simulink model "vector"  (R2025b)
settings: Solver=FixedStepAuto  StartTime=0.0  StopTime=30  FixedStep=0.05  RelTol=1e-3
undefined symbols (not defined in the file or in its folder): DiscIntNeverNeededParam
libraries: rllib x1
(part 1 of 2)
settings Model: Creator=heodo  LastModifiedBy=heodo

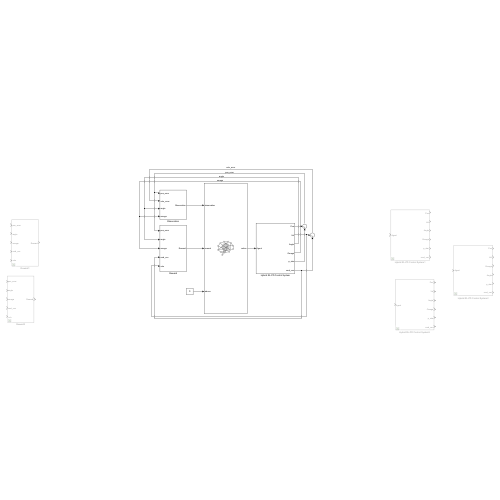
[thumbnail: Simulink's stored preview of the top-level diagram]
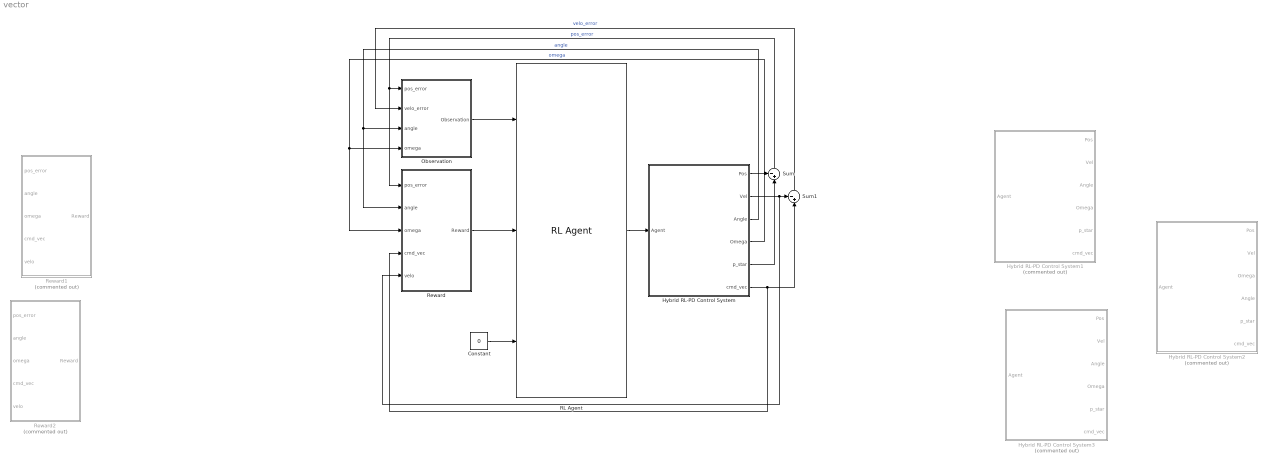
== system vector ==
  Constant : Constant  Value=0
  Hybrid RL-PD Control System : Subsystem
  Hybrid RL-PD Control System1 : Subsystem  Commented=on
  Hybrid RL-PD Control System2 : Subsystem  Commented=on
  Hybrid RL-PD Control System3 : Subsystem  Commented=on
  Observation : Subsystem
  RL Agent : rllib/RL Agent  Agent=agent  ExternalActionAsInput=off  ProvideLastAction=off  ProvideCumRwd=off  TreatAsDirectFeedthrough=on  UseStrictObservationDataTypes=off
  Reward : Subsystem
  Reward1 : Subsystem  Commented=on
  Reward2 : Subsystem  Commented=on
  Sum : Sum  Inputs=-+|
  Sum1 : Sum  Inputs=-+|
  wires:
  Observation/1(Observation) -> RL Agent/1
  Reward/1(Reward) -> RL Agent/2
  RL Agent/1 -> Hybrid RL-PD Control System/1(Agent)
  Hybrid RL-PD Control System/1(Pos) -> Sum/1
  Hybrid RL-PD Control System/5(p_star) -> Sum/2
  Sum/1 -> Reward/1(pos_error), Observation/1(pos_error)  "pos_error"
  Hybrid RL-PD Control System/2(Vel) -> Reward/5(velo), Sum1/1
  Hybrid RL-PD Control System/6(cmd_vec) -> Sum1/2, Reward/4(cmd_vec)
  Sum1/1 -> Observation/2(velo_error)  "velo_error"
  Hybrid RL-PD Control System/3(Angle) -> Observation/3(angle), Reward/2(angle)  "angle"
  Hybrid RL-PD Control System/4(Omega) -> Observation/4(omega), Reward/3(omega)  "omega"
  Constant/1 -> RL Agent/3

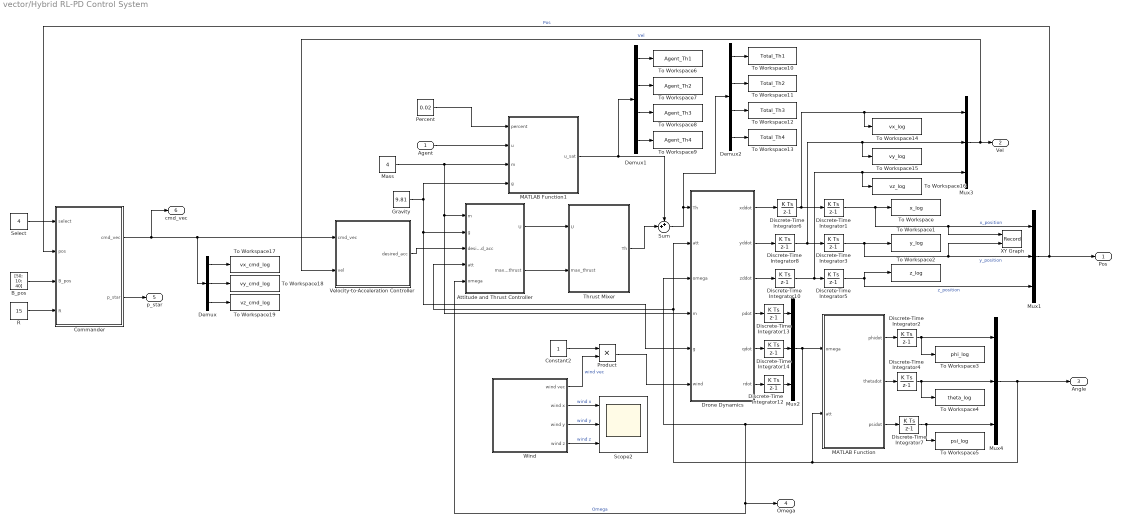
== system vector/Hybrid RL-PD Control System ==
  Agent : Inport
  Attitude and Thrust Controller : MATLAB Function  TreatAsAtomicUnit=on
  B_pos : Constant  Value=[50; 10; 40]
  Commander : MATLAB Function  TreatAsAtomicUnit=on
  Constant2 : Constant
  Demux : Demux  Outputs=3
  Demux1 : Demux
  Demux2 : Demux
  Discrete-Time Integrator{1..4,6..8,10,12..14} (11 alike) : DiscreteIntegrator  SampleTime=-1  ICPrevOutput=DiscIntNeverNeededParam  ICPrevScaledInput=DiscIntNeverNeededParam
  Discrete-Time Integrator5 : DiscreteIntegrator  InitialCondition=25  SampleTime=-1  ICPrevOutput=DiscIntNeverNeededParam  ICPrevScaledInput=DiscIntNeverNeededParam
  Drone Dynamics : MATLAB Function  TreatAsAtomicUnit=on
  Gravity : Constant  Value=9.81
  MATLAB Function : MATLAB Function  TreatAsAtomicUnit=on
  MATLAB Function1 : MATLAB Function  TreatAsAtomicUnit=on
  Mass : Constant  Value=4
  Mux{1..4} (4 alike) : Mux  Inputs=3
  Percent : Constant  Value=0.02
  Product : Product
  R : Constant  Value=15
  Scope2 : Scope  NumInputPorts=3
      settings: ActiveDisplayYMinimum=-12.935318443726832  ActiveDisplayYMaximum=12.935318443726839  DataLoggingVariableName=ScopeData2
  Select : Constant  Value=4
  Sum : Sum  Inputs=++|
  Thrust Mixer : MATLAB Function  TreatAsAtomicUnit=on
  To Workspace : ToWorkspace  VariableName=x_log  SaveFormat=Timeseries  SampleTime=-1
  To Workspace1 : ToWorkspace  VariableName=y_log  SaveFormat=Timeseries  SampleTime=-1
  To Workspace10 : ToWorkspace  VariableName=Total_Th1  SaveFormat=Timeseries  SampleTime=-1
  To Workspace11 : ToWorkspace  VariableName=Total_Th2  SaveFormat=Timeseries  SampleTime=-1
  To Workspace12 : ToWorkspace  VariableName=Total_Th3  SaveFormat=Timeseries  SampleTime=-1
  To Workspace13 : ToWorkspace  VariableName=Total_Th4  SaveFormat=Timeseries  SampleTime=-1
  To Workspace14 : ToWorkspace  VariableName=vx_log  SaveFormat=Timeseries  SampleTime=-1
  To Workspace15 : ToWorkspace  VariableName=vy_log  SaveFormat=Timeseries  SampleTime=-1
  To Workspace16 : ToWorkspace  VariableName=vz_log  SaveFormat=Timeseries  SampleTime=-1
  To Workspace17 : ToWorkspace  VariableName=vx_cmd_log  SaveFormat=Timeseries  SampleTime=-1
  To Workspace18 : ToWorkspace  VariableName=vy_cmd_log  SaveFormat=Timeseries  SampleTime=-1
  To Workspace19 : ToWorkspace  VariableName=vz_cmd_log  SaveFormat=Timeseries  SampleTime=-1
  To Workspace2 : ToWorkspace  VariableName=z_log  SaveFormat=Timeseries  SampleTime=-1
  To Workspace3 : ToWorkspace  VariableName=phi_log  SaveFormat=Timeseries  SampleTime=-1
  To Workspace4 : ToWorkspace  VariableName=theta_log  SaveFormat=Timeseries  SampleTime=-1
  To Workspace5 : ToWorkspace  VariableName=psi_log  SaveFormat=Timeseries  SampleTime=-1
  To Workspace6 : ToWorkspace  VariableName=Agent_Th1  SaveFormat=Timeseries  SampleTime=-1
  To Workspace7 : ToWorkspace  VariableName=Agent_Th2  SaveFormat=Timeseries  SampleTime=-1
  To Workspace8 : ToWorkspace  VariableName=Agent_Th3  SaveFormat=Timeseries  SampleTime=-1
  To Workspace9 : ToWorkspace  VariableName=Agent_Th4  SaveFormat=Timeseries  SampleTime=-1
  Velocity-to-Acceleration Controller : MATLAB Function  TreatAsAtomicUnit=on
  Wind : Subsystem
  XY Graph : Record  NumPorts=2.0  FileSettingsInternal="{\"entries\":[{\"content\":{\"excelSettings\":{\"content\":{},\"type\":\"Streamout.ExcelSettings\"},\"parquetSettings\":{\"content\":{},\"type\":\"Streamout.ParquetSettings\"}},\"type\":\"Streamout.FileSettingStorage\",\"uuid\":\"\"}],\"packageUris\":[\"http:\\/\\/schema.mathworks.com\\/mf0\\/streamout_blocks\\/R2020a\"],\"version\":\"1.0\"}"  FrameSettings=[0, 0]  Layout=[1 1]  SignalsInternal="{\"entries\":[{\"content\":{\"signals\":[{\"content\":{\"blockPath\":[],\"dimensions\":[1],\"domain\":\"\",\"lineColor\":\"#a2142f\",\"plots\":[ 1 ],\"port\":1,\"signalID\":1,\"signalName\":\"x_position\"},\"type\":\"RecordBlkView.Signal\",\"uuid\":\"\"},{\"content\":{\"blockPath\":[],\"dimensions\":[1],\"domain\":\"\",\"lineColor\":\"#139fff\",\"plots\":[ 1 ],\"port\":2,\"signalID\":2,\"signalName\":\"y_position\"},\"type\":\"RecordBlkView.Signal\",\"uuid\":\"\"}]},\"type\":\"RecordBlkView.InputSignals\",\"uuid\":\"\"}],\"packageUris\":[\"http:\\/\\/schema.mathworks.com\\/mf0\\/streamout_blocks\\/R2020a\"],\"version\":\"1.0\"}"  VisualizationBindings="{\"xyplotplugin\":{\"info\":[{\"series\":[{\"bindingParametersList\":[{\"parameter\":\"X-Axis\",\"signalID\":1,\"signalName\":\"x_position\"},{\"parameter\":\"Y-Axis\",\"signalID\":2,\"signalName\":\"y_position\"}],\"seriesID\":0}],\"subplotID\":1}]}}"  CompatibilityTag=XY
  Pos : Outport
  Vel : Outport  Port=2
  Angle : Outport  Port=3
  Omega : Outport  Port=4
  p_star : Outport  Port=5
  cmd_vec : Outport  Port=6
  wires:
  Velocity-to-Acceleration Controller/1(desired_acc) -> Attitude and Thrust Controller/3(desired_acc)
  Gravity/1 -> MATLAB Function1/4(g), Attitude and Thrust Controller/2(g), Drone Dynamics/5(g)
  Mass/1 -> Attitude and Thrust Controller/1(m), Drone Dynamics/4(m), MATLAB Function1/3(m)
  Attitude and Thrust Controller/1(U) -> Thrust Mixer/1(U)
  Attitude and Thrust Controller/2(max_thrust) -> Thrust Mixer/2(max_thrust)
  Mux4/1 -> MATLAB Function/2(att), Drone Dynamics/2(att), Attitude and Thrust Controller/4(att), Angle/1
  Discrete-Time Integrator5/1 -> To Workspace2/1, Mux1/3  "z_position"
  Discrete-Time Integrator1/1 -> XY Graph/1, Mux1/1, To Workspace/1  "x_position"
  Discrete-Time Integrator3/1 -> To Workspace1/1, XY Graph/2, Mux1/2  "y_position"
  Mux1/1 -> Pos/1, Commander/2(pos)  "Pos"
  Thrust Mixer/1(Th) -> Sum/2
  Sum/1 -> Demux2/1, Drone Dynamics/1(Th)
  Mux3/1 -> Vel/1, Velocity-to-Acceleration Controller/2(vel)  "Vel"
  Mux2/1 -> MATLAB Function/1(omega), Drone Dynamics/3(omega), Attitude and Thrust Controller/5(omega), Omega/1  "Omega"
  Demux1/1 -> To Workspace6/1
  Demux1/4 -> To Workspace9/1
  Demux1/3 -> To Workspace8/1
  Demux1/2 -> To Workspace7/1
  Demux2/3 -> To Workspace12/1
  Demux2/4 -> To Workspace13/1
  Demux2/2 -> To Workspace11/1
  Demux2/1 -> To Workspace10/1
  R/1 -> Commander/4(R)
  Select/1 -> Commander/1(select)
  B_pos/1 -> Commander/3(B_pos)
  Commander/1(cmd_vec) -> cmd_vec/1, Demux/1, Velocity-to-Acceleration Controller/1(cmd_vec)
  Commander/2(p_star) -> p_star/1
  Wind/2(wind x) -> Scope2/1  "wind x"
  Wind/3(wind y) -> Scope2/2  "wind y"
  Wind/4(wind z) -> Scope2/3  "wind z"
  Wind/1(wind vec) -> Product/2  "wind vec"
  Constant2/1 -> Product/1
  Product/1 -> Drone Dynamics/6(wind)
  Drone Dynamics/3(zddot) -> Discrete-Time Integrator10/1
  Drone Dynamics/2(yddot) -> Discrete-Time Integrator8/1
  Drone Dynamics/1(xddot) -> Discrete-Time Integrator6/1
  Discrete-Time Integrator6/1 -> Discrete-Time Integrator1/1, To Workspace14/1, Mux3/1
  Discrete-Time Integrator8/1 -> Discrete-Time Integrator3/1, To Workspace15/1, Mux3/2
  Discrete-Time Integrator10/1 -> To Workspace16/1, Mux3/3, Discrete-Time Integrator5/1
  Discrete-Time Integrator12/1 -> Mux2/3
  Drone Dynamics/6(rdot) -> Discrete-Time Integrator12/1
  Drone Dynamics/5(qdot) -> Discrete-Time Integrator14/1
  Discrete-Time Integrator14/1 -> Mux2/2
  Drone Dynamics/4(pdot) -> Discrete-Time Integrator13/1
  Discrete-Time Integrator13/1 -> Mux2/1
  MATLAB Function/1(phidot) -> Discrete-Time Integrator2/1
  MATLAB Function/2(thetadot) -> Discrete-Time Integrator4/1
  MATLAB Function/3(psidot) -> Discrete-Time Integrator7/1
  Discrete-Time Integrator2/1 -> Mux4/1, To Workspace3/1
  Discrete-Time Integrator4/1 -> To Workspace4/1, Mux4/2
  Discrete-Time Integrator7/1 -> To Workspace5/1, Mux4/3
  Demux/1 -> To Workspace17/1
  Demux/2 -> To Workspace18/1
  Demux/3 -> To Workspace19/1
  Agent/1 -> MATLAB Function1/2(u)
  MATLAB Function1/1(u_sat) -> Sum/1, Demux1/1
  Percent/1 -> MATLAB Function1/1(percent)

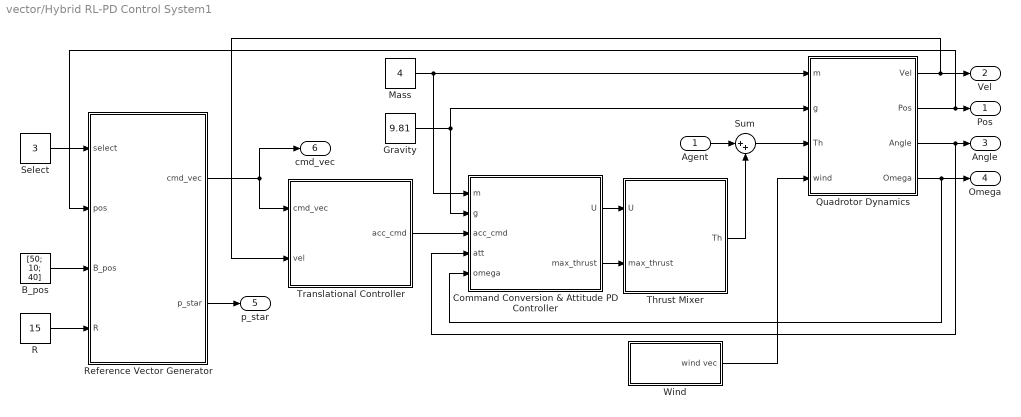
== system vector/Hybrid RL-PD Control System1 ==
  Agent : Inport
  B_pos : Constant  Value=[50; 10; 40]
  Command Conversion & Attitude PD Controller : MATLAB Function  TreatAsAtomicUnit=on
  Gravity : Constant  Value=9.81
  Mass : Constant  Value=4
  Quadrotor Dynamics : Subsystem
  R : Constant  Value=15
  Reference Vector Generator : MATLAB Function  TreatAsAtomicUnit=on
  Select : Constant  Value=3
  Sum : Sum  Inputs=|++
  Thrust Mixer : MATLAB Function  TreatAsAtomicUnit=on
  Translational Controller : MATLAB Function  TreatAsAtomicUnit=on
  Wind : Subsystem
  Pos : Outport
  Vel : Outport  Port=2
  Angle : Outport  Port=3
  Omega : Outport  Port=4
  p_star : Outport  Port=5
  cmd_vec : Outport  Port=6
  wires:
  Translational Controller/1(acc_cmd) -> Command Conversion & Attitude PD Controller/3(acc_cmd)
  Gravity/1 -> Quadrotor Dynamics/2(g), Command Conversion & Attitude PD Controller/2(g)
  Mass/1 -> Command Conversion & Attitude PD Controller/1(m), Quadrotor Dynamics/1(m)
  Command Conversion & Attitude PD Controller/1(U) -> Thrust Mixer/1(U)
  Command Conversion & Attitude PD Controller/2(max_thrust) -> Thrust Mixer/2(max_thrust)
  R/1 -> Reference Vector Generator/4(R)
  Select/1 -> Reference Vector Generator/1(select)
  B_pos/1 -> Reference Vector Generator/3(B_pos)
  Reference Vector Generator/1(cmd_vec) -> cmd_vec/1, Translational Controller/1(cmd_vec)
  Reference Vector Generator/2(p_star) -> p_star/1
  Sum/1 -> Quadrotor Dynamics/3(Th)
  Wind/1(wind vec) -> Quadrotor Dynamics/4(wind)
  Quadrotor Dynamics/1(Vel) -> Vel/1, Translational Controller/2(vel)
  Quadrotor Dynamics/3(Angle) -> Angle/1, Command Conversion & Attitude PD Controller/4(att)
  Quadrotor Dynamics/4(Omega) -> Omega/1, Command Conversion & Attitude PD Controller/5(omega)
  Quadrotor Dynamics/2(Pos) -> Pos/1, Reference Vector Generator/2(pos)
  Agent/1 -> Sum/1
  Thrust Mixer/1(Th) -> Sum/2

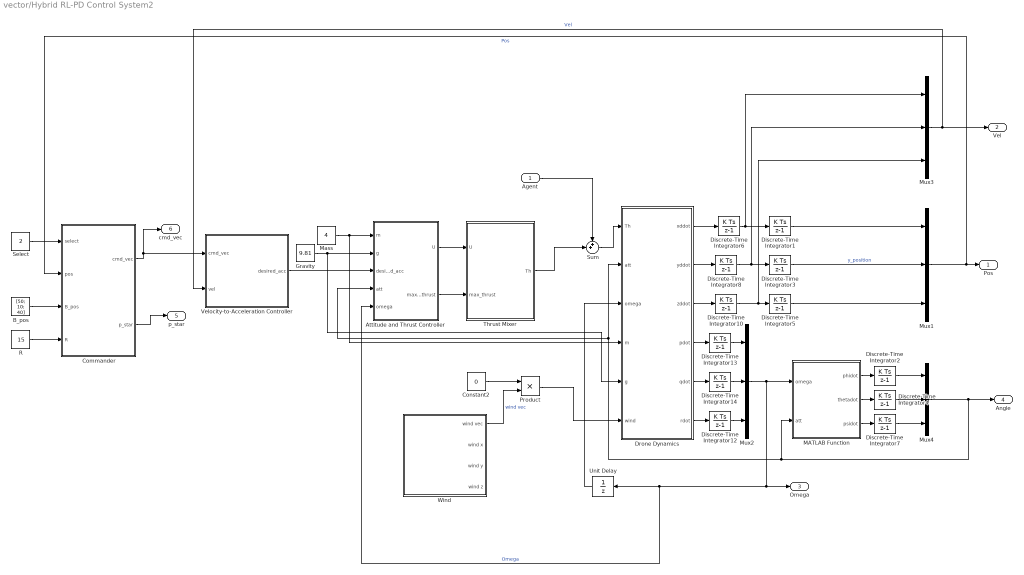
== system vector/Hybrid RL-PD Control System2 ==
  Agent : Inport
  Attitude and Thrust Controller : MATLAB Function  TreatAsAtomicUnit=on
  B_pos : Constant  Value=[50; 10; 40]
  Commander : MATLAB Function  TreatAsAtomicUnit=on
  Constant2 : Constant  Value=0
  Discrete-Time Integrator{1..4,7,12..14} (8 alike) : DiscreteIntegrator  SampleTime=-1  ICPrevOutput=DiscIntNeverNeededParam  ICPrevScaledInput=DiscIntNeverNeededParam
  Discrete-Time Integrator{5..6,8,10} (4 alike) : DiscreteIntegrator  InitialCondition=25  SampleTime=-1  ICPrevOutput=DiscIntNeverNeededParam  ICPrevScaledInput=DiscIntNeverNeededParam
  Drone Dynamics : MATLAB Function  TreatAsAtomicUnit=on
  Gravity : Constant  Value=9.81
  MATLAB Function : MATLAB Function  TreatAsAtomicUnit=on
  Mass : Constant  Value=4
  Mux{1..4} (4 alike) : Mux  Inputs=3
  Product : Product
  R : Constant  Value=15
  Select : Constant  Value=2
  Sum : Sum  Inputs=++|
  Thrust Mixer : MATLAB Function  TreatAsAtomicUnit=on
  Unit Delay : UnitDelay  SampleTime=-1  HasFrameUpgradeWarning=on
  Velocity-to-Acceleration Controller : MATLAB Function  TreatAsAtomicUnit=on
  Wind : Subsystem
  Pos : Outport
  Vel : Outport  Port=2
  Omega : Outport  Port=3
  Angle : Outport  Port=4
  p_star : Outport  Port=5
  cmd_vec : Outport  Port=6
  wires:
  Velocity-to-Acceleration Controller/1(desired_acc) -> Attitude and Thrust Controller/3(desired_acc)
  Gravity/1 -> Attitude and Thrust Controller/2(g), Drone Dynamics/5(g)
  Mass/1 -> Attitude and Thrust Controller/1(m), Drone Dynamics/4(m)
  Attitude and Thrust Controller/1(U) -> Thrust Mixer/1(U)
  Attitude and Thrust Controller/2(max_thrust) -> Thrust Mixer/2(max_thrust)
  Mux4/1 -> Angle/1, Drone Dynamics/2(att), Attitude and Thrust Controller/4(att), MATLAB Function/2(att)
  Discrete-Time Integrator5/1 -> Mux1/3
  Discrete-Time Integrator1/1 -> Mux1/1
  Discrete-Time Integrator3/1 -> Mux1/2  "y_position"
  Mux1/1 -> Pos/1, Commander/2(pos)  "Pos"
  Thrust Mixer/1(Th) -> Sum/2
  Sum/1 -> Drone Dynamics/1(Th)
  Mux3/1 -> Velocity-to-Acceleration Controller/2(vel), Vel/1  "Vel"
  Mux2/1 -> Attitude and Thrust Controller/5(omega), Unit Delay/1, Omega/1, MATLAB Function/1(omega)  "Omega"
  Agent/1 -> Sum/1
  R/1 -> Commander/4(R)
  Select/1 -> Commander/1(select)
  B_pos/1 -> Commander/3(B_pos)
  Commander/1(cmd_vec) -> cmd_vec/1, Velocity-to-Acceleration Controller/1(cmd_vec)
  Commander/2(p_star) -> p_star/1
  Wind/1(wind vec) -> Product/2  "wind vec"
  Constant2/1 -> Product/1
  Product/1 -> Drone Dynamics/6(wind)
  Drone Dynamics/3(zddot) -> Discrete-Time Integrator10/1
  Drone Dynamics/2(yddot) -> Discrete-Time Integrator8/1
  Drone Dynamics/1(xddot) -> Discrete-Time Integrator6/1
  Discrete-Time Integrator6/1 -> Discrete-Time Integrator1/1, Mux3/1
  Discrete-Time Integrator8/1 -> Discrete-Time Integrator3/1, Mux3/2
  Discrete-Time Integrator10/1 -> Mux3/3, Discrete-Time Integrator5/1
  Discrete-Time Integrator12/1 -> Mux2/3
  Drone Dynamics/6(rdot) -> Discrete-Time Integrator12/1
  Drone Dynamics/5(qdot) -> Discrete-Time Integrator14/1
  Discrete-Time Integrator14/1 -> Mux2/2
  Drone Dynamics/4(pdot) -> Discrete-Time Integrator13/1
  Discrete-Time Integrator13/1 -> Mux2/1
  Unit Delay/1 -> Drone Dynamics/3(omega)
  MATLAB Function/1(phidot) -> Discrete-Time Integrator2/1
  MATLAB Function/2(thetadot) -> Discrete-Time Integrator4/1
  MATLAB Function/3(psidot) -> Discrete-Time Integrator7/1
  Discrete-Time Integrator2/1 -> Mux4/1
  Discrete-Time Integrator4/1 -> Mux4/2
  Discrete-Time Integrator7/1 -> Mux4/3

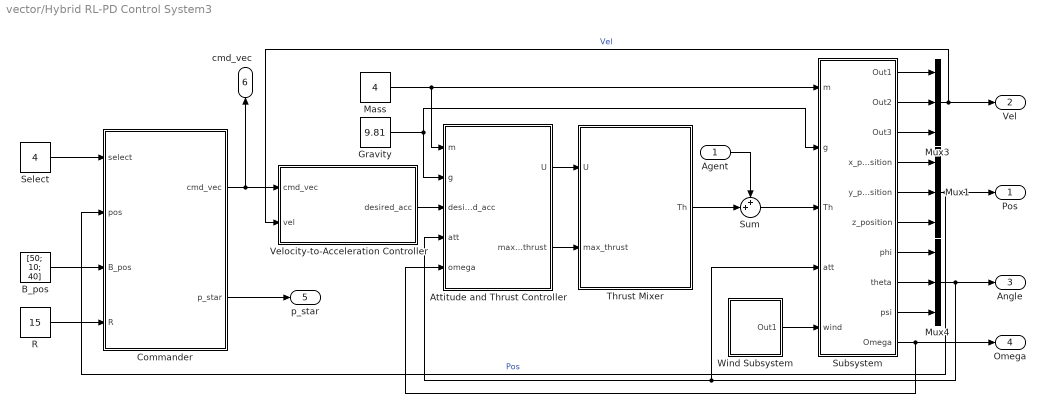
== system vector/Hybrid RL-PD Control System3 ==
  Agent : Inport
  Attitude and Thrust Controller : MATLAB Function  TreatAsAtomicUnit=on
  B_pos : Constant  Value=[50; 10; 40]
  Commander : MATLAB Function  TreatAsAtomicUnit=on
  Gravity : Constant  Value=9.81
  Mass : Constant  Value=4
  Mux1 : Mux  Inputs=3
  Mux3 : Mux  Inputs=3
  Mux4 : Mux  Inputs=3
  R : Constant  Value=15
  Select : Constant  Value=4
  Subsystem : Subsystem
  Sum : Sum  Inputs=++|
  Thrust Mixer : MATLAB Function  TreatAsAtomicUnit=on
  Velocity-to-Acceleration Controller : MATLAB Function  TreatAsAtomicUnit=on
  Wind Subsystem : Subsystem
  Pos : Outport
  Vel : Outport  Port=2
  Angle : Outport  Port=3
  Omega : Outport  Port=4
  p_star : Outport  Port=5
  cmd_vec : Outport  Port=6
  wires:
  Velocity-to-Acceleration Controller/1(desired_acc) -> Attitude and Thrust Controller/3(desired_acc)
  Gravity/1 -> Attitude and Thrust Controller/2(g), Subsystem/2(g)
  Mass/1 -> Attitude and Thrust Controller/1(m), Subsystem/1(m)
  Attitude and Thrust Controller/1(U) -> Thrust Mixer/1(U)
  Attitude and Thrust Controller/2(max_thrust) -> Thrust Mixer/2(max_thrust)
  Mux4/1 -> Angle/1, Attitude and Thrust Controller/4(att), Subsystem/4(att)
  Mux1/1 -> Pos/1, Commander/2(pos)  "Pos"
  Thrust Mixer/1(Th) -> Sum/2
  Mux3/1 -> Vel/1, Velocity-to-Acceleration Controller/2(vel)  "Vel"
  Agent/1 -> Sum/1
  R/1 -> Commander/4(R)
  Select/1 -> Commander/1(select)
  B_pos/1 -> Commander/3(B_pos)
  Commander/1(cmd_vec) -> Velocity-to-Acceleration Controller/1(cmd_vec), cmd_vec/1
  Commander/2(p_star) -> p_star/1
  Subsystem/10(Omega) -> Attitude and Thrust Controller/5(omega), Omega/1
  Sum/1 -> Subsystem/3(Th)
  Wind Subsystem/1(Out1) -> Subsystem/5(wind)
  Subsystem/1(Out1) -> Mux3/1
  Subsystem/2(Out2) -> Mux3/2
  Subsystem/3(Out3) -> Mux3/3
  Subsystem/4(x_position) -> Mux1/1
  Subsystem/5(y_position) -> Mux1/2
  Subsystem/6(z_position) -> Mux1/3
  Subsystem/7(phi) -> Mux4/1
  Subsystem/8(theta) -> Mux4/2
  Subsystem/9(psi) -> Mux4/3

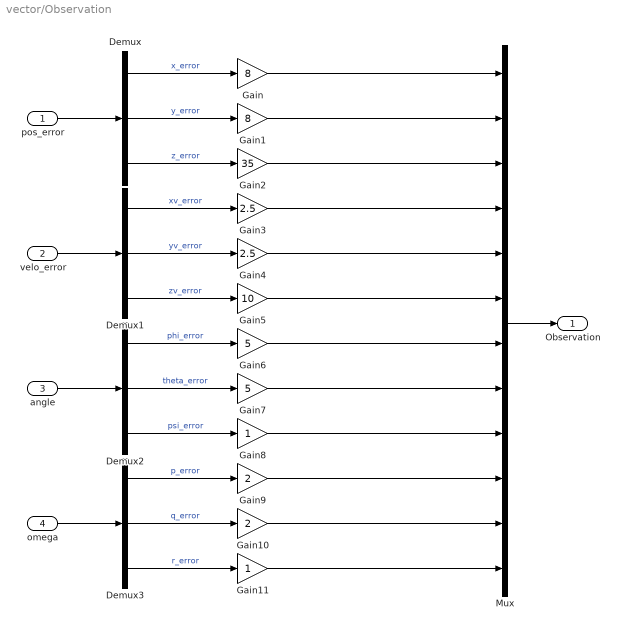
== system vector/Observation ==
  pos_error : Inport
  velo_error : Inport  Port=2
  angle : Inport  Port=3
  omega : Inport  Port=4
  Demux{,1..3} (4 alike) : Demux  Outputs=3
  Gain : Gain  Gain=8
  Gain1 : Gain  Gain=8
  Gain10 : Gain  Gain=2
  Gain11 : Gain
  Gain2 : Gain  Gain=35
  Gain3 : Gain  Gain=2.5
  Gain4 : Gain  Gain=2.5
  Gain5 : Gain  Gain=10
  Gain6 : Gain  Gain=5
  Gain7 : Gain  Gain=5
  Gain8 : Gain
  Gain9 : Gain  Gain=2
  Mux : Mux  Inputs=12
  Observation : Outport
  wires:
  Mux/1 -> Observation/1
  Demux/1 -> Gain/1  "x_error"
  Demux/2 -> Gain1/1  "y_error"
  Demux/3 -> Gain2/1  "z_error"
  Demux1/2 -> Gain4/1  "yv_error"
  Demux1/1 -> Gain3/1  "xv_error"
  Demux1/3 -> Gain5/1  "zv_error"
  Demux2/2 -> Gain7/1  "theta_error"
  Demux2/1 -> Gain6/1  "phi_error"
  Demux2/3 -> Gain8/1  "psi_error"
  Demux3/2 -> Gain10/1  "q_error"
  Demux3/1 -> Gain9/1  "p_error"
  Demux3/3 -> Gain11/1  "r_error"
  omega/1 -> Demux3/1
  angle/1 -> Demux2/1
  velo_error/1 -> Demux1/1
  pos_error/1 -> Demux/1
  Gain/1 -> Mux/1
  Gain1/1 -> Mux/2
  Gain2/1 -> Mux/3
  Gain3/1 -> Mux/4
  Gain4/1 -> Mux/5
  Gain5/1 -> Mux/6
  Gain6/1 -> Mux/7
  Gain7/1 -> Mux/8
  Gain8/1 -> Mux/9
  Gain9/1 -> Mux/10
  Gain10/1 -> Mux/11
  Gain11/1 -> Mux/12

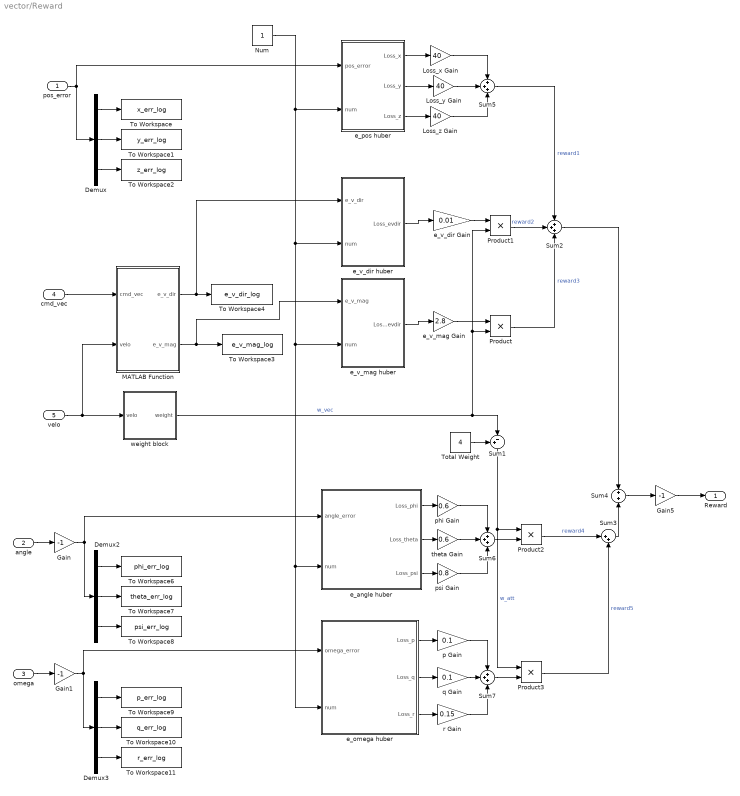
== system vector/Reward ==
  pos_error : Inport
  angle : Inport  Port=2
  omega : Inport  Port=3
  cmd_vec : Inport  Port=4
  velo : Inport  Port=5
  " e_angle huber" : MATLAB Function  TreatAsAtomicUnit=on
  Demux : Demux  Outputs=3
  Demux2 : Demux  Outputs=3
  Demux3 : Demux  Outputs=3
  Gain : Gain  Gain=-1
  Gain1 : Gain  Gain=-1
  Gain5 : Gain  Gain=-1
  Loss_x Gain : Gain  Gain=40
  Loss_y Gain : Gain  Gain=40
  Loss_z Gain : Gain  Gain=40
  MATLAB Function : MATLAB Function  TreatAsAtomicUnit=on
  Num : Constant
  Product{,1..3} (4 alike) : Product
  Sum1 : Sum  Inputs=+-|
  Sum{2,5..7} (4 alike) : Sum  Inputs=+++
  Sum3 : Sum  Inputs=|++
  Sum4 : Sum  Inputs=+|+
  To Workspace : ToWorkspace  VariableName=x_err_log  SaveFormat=Timeseries  SampleTime=-1
  To Workspace1 : ToWorkspace  VariableName=y_err_log  SaveFormat=Timeseries  SampleTime=-1
  To Workspace10 : ToWorkspace  VariableName=q_err_log  SaveFormat=Timeseries  SampleTime=-1
  To Workspace11 : ToWorkspace  VariableName=r_err_log  SaveFormat=Timeseries  SampleTime=-1
  To Workspace2 : ToWorkspace  VariableName=z_err_log  SaveFormat=Timeseries  SampleTime=-1
  To Workspace3 : ToWorkspace  VariableName=e_v_mag_log  SaveFormat=Timeseries  SampleTime=-1
  To Workspace4 : ToWorkspace  VariableName=e_v_dir_log  SaveFormat=Timeseries  SampleTime=-1
  To Workspace6 : ToWorkspace  VariableName=phi_err_log  SaveFormat=Timeseries  SampleTime=-1
  To Workspace7 : ToWorkspace  VariableName=theta_err_log  SaveFormat=Timeseries  SampleTime=-1
  To Workspace8 : ToWorkspace  VariableName=psi_err_log  SaveFormat=Timeseries  SampleTime=-1
  To Workspace9 : ToWorkspace  VariableName=p_err_log  SaveFormat=Timeseries  SampleTime=-1
  Total Weight : Constant  Value=4
  e_omega huber : MATLAB Function  TreatAsAtomicUnit=on
  e_pos huber : MATLAB Function  TreatAsAtomicUnit=on
  e_v_dir Gain : Gain  Gain=0.01
  e_v_dir huber : MATLAB Function  TreatAsAtomicUnit=on
  e_v_mag Gain : Gain  Gain=2.8
  e_v_mag huber : MATLAB Function  TreatAsAtomicUnit=on
  p Gain : Gain  Gain=0.1
  phi Gain : Gain  Gain=0.6
  psi Gain : Gain  Gain=0.8
  q Gain : Gain  Gain=0.1
  r Gain : Gain  Gain=0.15
  theta Gain : Gain  Gain=0.6
  weight block : Subsystem
  Reward : Outport
  wires:
  pos_error/1 -> Demux/1, e_pos huber/1(pos_error)
  Gain5/1 -> Reward/1
  Demux/1 -> To Workspace/1
  Demux/2 -> To Workspace1/1
  Demux/3 -> To Workspace2/1
  MATLAB Function/1(e_v_dir) -> To Workspace4/1, e_v_dir huber/1(e_v_dir)
  Demux2/3 -> To Workspace8/1
  Demux2/1 -> To Workspace6/1
  Demux2/2 -> To Workspace7/1
  angle/1 -> Gain/1
  Demux3/3 -> To Workspace11/1
  Demux3/1 -> To Workspace9/1
  Demux3/2 -> To Workspace10/1
  omega/1 -> Gain1/1
  velo/1 -> MATLAB Function/2(velo), weight block/1(velo)
  Gain/1 -> Demux2/1, " e_angle huber"/1(angle_error)
  Gain1/1 -> Demux3/1, e_omega huber/1(omega_error)
  cmd_vec/1 -> MATLAB Function/1(cmd_vec)
  e_v_mag huber/1(Loss_evdir) -> e_v_mag Gain/1
  e_v_mag Gain/1 -> Product/1
  MATLAB Function/2(e_v_mag) -> To Workspace3/1, e_v_mag huber/1(e_v_mag)
  e_v_dir huber/1(Loss_evdir) -> e_v_dir Gain/1
  e_v_dir Gain/1 -> Product1/1
  Total Weight/1 -> Sum1/1
  Sum1/1 -> Product3/1, Product2/1  "w_att"
  e_pos huber/1(Loss_x) -> Loss_x Gain/1
  Product1/1 -> Sum2/2  "reward2"
  Product/1 -> Sum2/3  "reward3"
  Product2/1 -> Sum3/1  "reward4"
  Product3/1 -> Sum3/2  "reward5"
  Sum3/1 -> Sum4/2
  Sum2/1 -> Sum4/1
  Sum4/1 -> Gain5/1
  weight block/1(weight) -> Product1/2, Product/2, Sum1/2  "w_vec"
  Loss_x Gain/1 -> Sum5/1
  e_pos huber/2(Loss_y) -> Loss_y Gain/1
  Loss_y Gain/1 -> Sum5/2
  e_pos huber/3(Loss_z) -> Loss_z Gain/1
  Loss_z Gain/1 -> Sum5/3
  Sum5/1 -> Sum2/1  "reward1"
  theta Gain/1 -> Sum6/2
  " e_angle huber"/1(Loss_phi) -> phi Gain/1
  " e_angle huber"/2(Loss_theta) -> theta Gain/1
  " e_angle huber"/3(Loss_psi) -> psi Gain/1
  psi Gain/1 -> Sum6/3
  phi Gain/1 -> Sum6/1
  Sum6/1 -> Product2/2
  r Gain/1 -> Sum7/3
  p Gain/1 -> Sum7/1
  Sum7/1 -> Product3/2
  q Gain/1 -> Sum7/2
  e_omega huber/1(Loss_p) -> p Gain/1
  e_omega huber/2(Loss_q) -> q Gain/1
  e_omega huber/3(Loss_r) -> r Gain/1
  Num/1 -> e_pos huber/2(num), e_v_dir huber/2(num), e_v_mag huber/2(num), " e_angle huber"/2(num), e_omega huber/2(num)

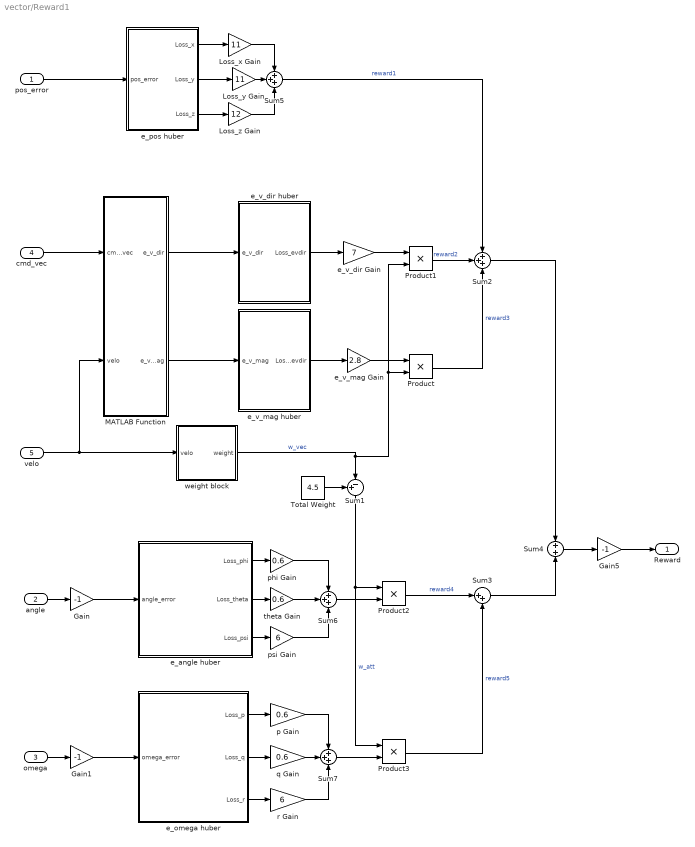
== system vector/Reward1 ==
  pos_error : Inport
  angle : Inport  Port=2
  omega : Inport  Port=3
  cmd_vec : Inport  Port=4
  velo : Inport  Port=5
  " e_angle huber" : MATLAB Function  TreatAsAtomicUnit=on
  Gain : Gain  Gain=-1
  Gain1 : Gain  Gain=-1
  Gain5 : Gain  Gain=-1
  Loss_x Gain : Gain  Gain=11
  Loss_y Gain : Gain  Gain=11
  Loss_z Gain : Gain  Gain=12
  MATLAB Function : MATLAB Function  TreatAsAtomicUnit=on
  Product{,1..3} (4 alike) : Product
  Sum1 : Sum  Inputs=+-|
  Sum{2,5..7} (4 alike) : Sum  Inputs=+++
  Sum3 : Sum  Inputs=|++
  Sum4 : Sum  Inputs=+|+
  Total Weight : Constant  Value=4.5
  e_omega huber : MATLAB Function  TreatAsAtomicUnit=on
  e_pos huber : MATLAB Function  TreatAsAtomicUnit=on
  e_v_dir Gain : Gain  Gain=7
  e_v_dir huber : MATLAB Function  TreatAsAtomicUnit=on
  e_v_mag Gain : Gain  Gain=2.8
  e_v_mag huber : MATLAB Function  TreatAsAtomicUnit=on
  p Gain : Gain  Gain=0.6
  phi Gain : Gain  Gain=0.6
  psi Gain : Gain  Gain=6
  q Gain : Gain  Gain=0.6
  r Gain : Gain  Gain=6
  theta Gain : Gain  Gain=0.6
  weight block : Subsystem
  Reward : Outport
  wires:
  pos_error/1 -> e_pos huber/1(pos_error)
  Gain5/1 -> Reward/1
  MATLAB Function/1(e_v_dir) -> e_v_dir huber/1(e_v_dir)
  angle/1 -> Gain/1
  omega/1 -> Gain1/1
  velo/1 -> weight block/1(velo), MATLAB Function/2(velo)
  Gain/1 -> " e_angle huber"/1(angle_error)
  Gain1/1 -> e_omega huber/1(omega_error)
  cmd_vec/1 -> MATLAB Function/1(cmd_vec)
  e_v_mag huber/1(Loss_evdir) -> e_v_mag Gain/1
  e_v_mag Gain/1 -> Product/1
  MATLAB Function/2(e_v_mag) -> e_v_mag huber/1(e_v_mag)
  e_v_dir huber/1(Loss_evdir) -> e_v_dir Gain/1
  e_v_dir Gain/1 -> Product1/1
  Total Weight/1 -> Sum1/1
  Sum1/1 -> Product3/1, Product2/1  "w_att"
  e_pos huber/1(Loss_x) -> Loss_x Gain/1
  Product1/1 -> Sum2/2  "reward2"
  Product/1 -> Sum2/3  "reward3"
  Product2/1 -> Sum3/1  "reward4"
  Product3/1 -> Sum3/2  "reward5"
  Sum3/1 -> Sum4/2
  Sum2/1 -> Sum4/1
  Sum4/1 -> Gain5/1
  weight block/1(weight) -> Product1/2, Product/2, Sum1/2  "w_vec"
  Loss_x Gain/1 -> Sum5/1
  e_pos huber/2(Loss_y) -> Loss_y Gain/1
  Loss_y Gain/1 -> Sum5/2
  e_pos huber/3(Loss_z) -> Loss_z Gain/1
  Loss_z Gain/1 -> Sum5/3
  Sum5/1 -> Sum2/1  "reward1"
  theta Gain/1 -> Sum6/2
  " e_angle huber"/1(Loss_phi) -> phi Gain/1
  " e_angle huber"/2(Loss_theta) -> theta Gain/1
  " e_angle huber"/3(Loss_psi) -> psi Gain/1
  psi Gain/1 -> Sum6/3
  phi Gain/1 -> Sum6/1
  Sum6/1 -> Product2/2
  r Gain/1 -> Sum7/3
  p Gain/1 -> Sum7/1
  Sum7/1 -> Product3/2
  q Gain/1 -> Sum7/2
  e_omega huber/1(Loss_p) -> p Gain/1
  e_omega huber/2(Loss_q) -> q Gain/1
  e_omega huber/3(Loss_r) -> r Gain/1

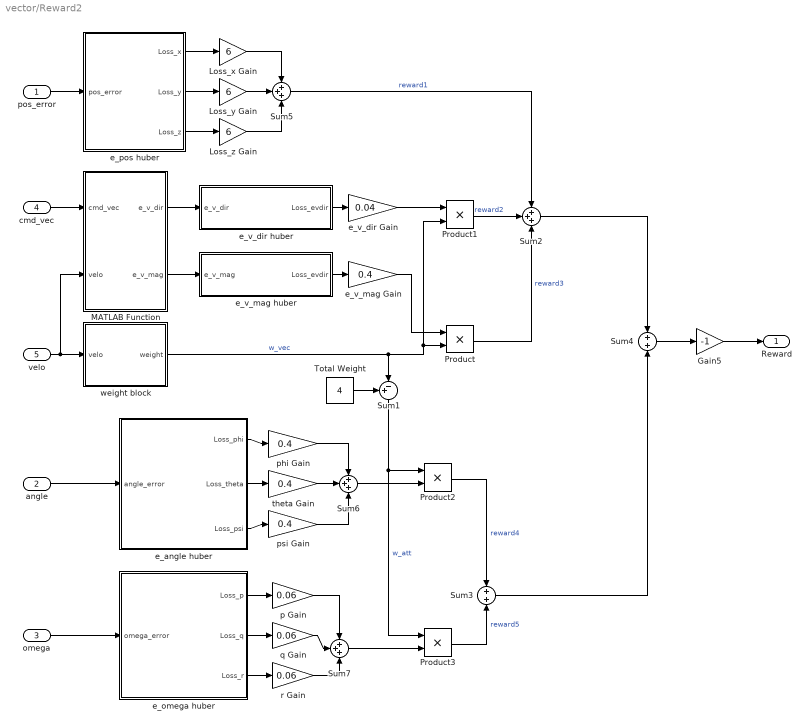
== system vector/Reward2 ==
  pos_error : Inport
  angle : Inport  Port=2
  omega : Inport  Port=3
  cmd_vec : Inport  Port=4
  velo : Inport  Port=5
  " e_angle huber" : MATLAB Function  TreatAsAtomicUnit=on
  Gain5 : Gain  Gain=-1
  Loss_x Gain : Gain  Gain=6
  Loss_y Gain : Gain  Gain=6
  Loss_z Gain : Gain  Gain=6
  MATLAB Function : MATLAB Function  TreatAsAtomicUnit=on
  Product{,1..3} (4 alike) : Product
  Sum1 : Sum  Inputs=+-|
  Sum{2,5..7} (4 alike) : Sum  Inputs=+++
  Sum3 : Sum  Inputs=+|+
  Sum4 : Sum  Inputs=+|+
  Total Weight : Constant  Value=4
  e_omega huber : MATLAB Function  TreatAsAtomicUnit=on
  e_pos huber : MATLAB Function  TreatAsAtomicUnit=on
  e_v_dir Gain : Gain  Gain=0.04
  e_v_dir huber : MATLAB Function  TreatAsAtomicUnit=on
  e_v_mag Gain : Gain  Gain=0.4
  e_v_mag huber : MATLAB Function  TreatAsAtomicUnit=on
  p Gain : Gain  Gain=0.06
  phi Gain : Gain  Gain=0.4
  psi Gain : Gain  Gain=0.4
  q Gain : Gain  Gain=0.06
  r Gain : Gain  Gain=0.06
  theta Gain : Gain  Gain=0.4
  weight block : Subsystem
  Reward : Outport
  wires:
  pos_error/1 -> e_pos huber/1(pos_error)
  Gain5/1 -> Reward/1
  MATLAB Function/1(e_v_dir) -> e_v_dir huber/1(e_v_dir)
  velo/1 -> MATLAB Function/2(velo), weight block/1(velo)
  angle/1 -> " e_angle huber"/1(angle_error)
  omega/1 -> e_omega huber/1(omega_error)
  cmd_vec/1 -> MATLAB Function/1(cmd_vec)
  e_v_mag huber/1(Loss_evdir) -> e_v_mag Gain/1
  e_v_mag Gain/1 -> Product/1
  MATLAB Function/2(e_v_mag) -> e_v_mag huber/1(e_v_mag)
  e_v_dir huber/1(Loss_evdir) -> e_v_dir Gain/1
  e_v_dir Gain/1 -> Product1/1
  Total Weight/1 -> Sum1/1
  Sum1/1 -> Product2/1, Product3/1  "w_att"
  e_pos huber/1(Loss_x) -> Loss_x Gain/1
  Product1/1 -> Sum2/2  "reward2"
  Product/1 -> Sum2/3  "reward3"
  Product2/1 -> Sum3/1  "reward4"
  Product3/1 -> Sum3/2  "reward5"
  Sum3/1 -> Sum4/2
  Sum2/1 -> Sum4/1
  Sum4/1 -> Gain5/1
  weight block/1(weight) -> Product/2, Product1/2, Sum1/2  "w_vec"
  Loss_x Gain/1 -> Sum5/1
  e_pos huber/2(Loss_y) -> Loss_y Gain/1
  Loss_y Gain/1 -> Sum5/2
  e_pos huber/3(Loss_z) -> Loss_z Gain/1
  Loss_z Gain/1 -> Sum5/3
  Sum5/1 -> Sum2/1  "reward1"
  theta Gain/1 -> Sum6/2
  " e_angle huber"/1(Loss_phi) -> phi Gain/1
  " e_angle huber"/2(Loss_theta) -> theta Gain/1
  " e_angle huber"/3(Loss_psi) -> psi Gain/1
  psi Gain/1 -> Sum6/3
  phi Gain/1 -> Sum6/1
  Sum6/1 -> Product2/2
  r Gain/1 -> Sum7/3
  p Gain/1 -> Sum7/1
  Sum7/1 -> Product3/2
  q Gain/1 -> Sum7/2
  e_omega huber/1(Loss_p) -> p Gain/1
  e_omega huber/2(Loss_q) -> q Gain/1
  e_omega huber/3(Loss_r) -> r Gain/1

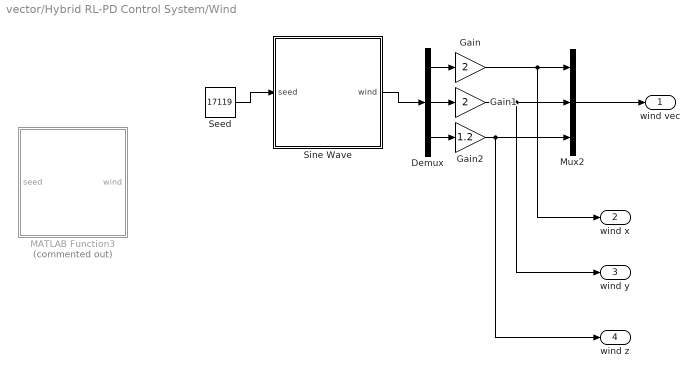
== system vector/Hybrid RL-PD Control System/Wind ==
  Demux : Demux  Outputs=3
  Gain : Gain  Gain=2
  Gain1 : Gain  Gain=2
  Gain2 : Gain  Gain=1.2
  MATLAB Function3 : MATLAB Function  Commented=on  TreatAsAtomicUnit=on
  Mux2 : Mux  Inputs=3
  Seed : Constant  Value=17119
  Sine Wave : MATLAB Function  TreatAsAtomicUnit=on
  wind vec : Outport
  wind x : Outport  Port=2
  wind y : Outport  Port=3
  wind z : Outport  Port=4
  wires:
  Demux/2 -> Gain1/1
  Gain1/1 -> wind y/1, Mux2/2
  Gain2/1 -> wind z/1, Mux2/3
  Demux/1 -> Gain/1
  Demux/3 -> Gain2/1
  Gain/1 -> wind x/1, Mux2/1
  Mux2/1 -> wind vec/1
  Seed/1 -> Sine Wave/1(seed)
  Sine Wave/1(wind) -> Demux/1

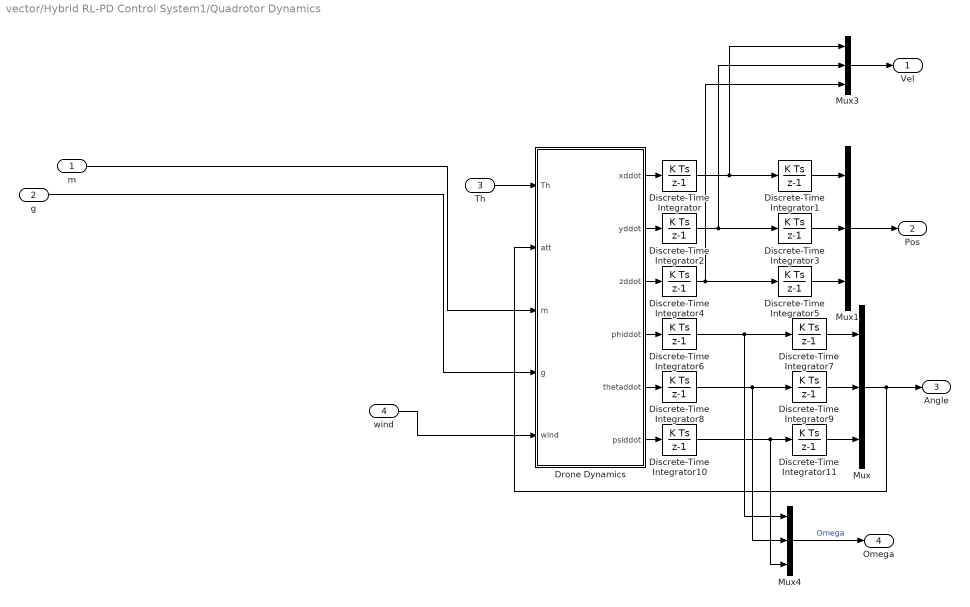
== system vector/Hybrid RL-PD Control System1/Quadrotor Dynamics ==
  m : Inport
  g : Inport  Port=2
  Th : Inport  Port=3
  wind : Inport  Port=4
  Discrete-Time Integrator{,1..4,6..11} (11 alike) : DiscreteIntegrator  SampleTime=-1  ICPrevOutput=DiscIntNeverNeededParam  ICPrevScaledInput=DiscIntNeverNeededParam
  Discrete-Time Integrator5 : DiscreteIntegrator  InitialCondition=25  SampleTime=-1  ICPrevOutput=DiscIntNeverNeededParam  ICPrevScaledInput=DiscIntNeverNeededParam
  Drone Dynamics : MATLAB Function  TreatAsAtomicUnit=on
  Mux{,1,3..4} (4 alike) : Mux  Inputs=3
  Vel : Outport
  Pos : Outport  Port=2
  Angle : Outport  Port=3
  Omega : Outport  Port=4
  wires:
  m/1 -> Drone Dynamics/3(m)
  Mux1/1 -> Pos/1
  Mux3/1 -> Vel/1
  Discrete-Time Integrator/1 -> Discrete-Time Integrator1/1, Mux3/1
  Discrete-Time Integrator5/1 -> Mux1/3
  Discrete-Time Integrator8/1 -> Mux4/2, Discrete-Time Integrator9/1
  Discrete-Time Integrator4/1 -> Discrete-Time Integrator5/1, Mux3/3
  Mux/1 -> Angle/1, Drone Dynamics/2(att)
  g/1 -> Drone Dynamics/4(g)
  Discrete-Time Integrator2/1 -> Discrete-Time Integrator3/1, Mux3/2
  Discrete-Time Integrator7/1 -> Mux/1
  Drone Dynamics/2(yddot) -> Discrete-Time Integrator2/1
  Discrete-Time Integrator3/1 -> Mux1/2
  Discrete-Time Integrator10/1 -> Mux4/3, Discrete-Time Integrator11/1
  Discrete-Time Integrator11/1 -> Mux/3
  Drone Dynamics/6(psiddot) -> Discrete-Time Integrator10/1
  Discrete-Time Integrator1/1 -> Mux1/1
  Discrete-Time Integrator9/1 -> Mux/2
  Drone Dynamics/4(phiddot) -> Discrete-Time Integrator6/1
  Drone Dynamics/5(thetaddot) -> Discrete-Time Integrator8/1
  Discrete-Time Integrator6/1 -> Mux4/1, Discrete-Time Integrator7/1
  Drone Dynamics/3(zddot) -> Discrete-Time Integrator4/1
  Drone Dynamics/1(xddot) -> Discrete-Time Integrator/1
  Mux4/1 -> Omega/1  "Omega"
  wind/1 -> Drone Dynamics/5(wind)
  Th/1 -> Drone Dynamics/1(Th)

== system vector/Hybrid RL-PD Control System1/Wind ==
  Demux : Demux  Outputs=3
  Gain : Gain  Gain=2
  Gain1 : Gain  Gain=2
  Gain2 : Gain  Gain=0.6
  MATLAB Function3 : MATLAB Function  TreatAsAtomicUnit=on
  Mux2 : Mux  Inputs=3
  Seed : Constant  Value=17119
  wind vec : Outport
  wires:
  Demux/2 -> Gain1/1
  Seed/1 -> MATLAB Function3/1(seed)
  Gain1/1 -> Mux2/2
  Gain2/1 -> Mux2/3
  Demux/1 -> Gain/1
  Demux/3 -> Gain2/1
  MATLAB Function3/1(wind) -> Demux/1
  Gain/1 -> Mux2/1
  Mux2/1 -> wind vec/1

== system vector/Hybrid RL-PD Control System2/Wind ==
  Demux : Demux  Outputs=3
  Gain : Gain  Gain=2
  Gain1 : Gain  Gain=2
  Gain2 : Gain  Gain=1.2
  MATLAB Function3 : MATLAB Function  TreatAsAtomicUnit=on
  Mux2 : Mux  Inputs=3
  Seed : Constant  Value=15762
  wind vec : Outport
  wind x : Outport  Port=2
  wind y : Outport  Port=3
  wind z : Outport  Port=4
  wires:
  Demux/2 -> Gain1/1
  Seed/1 -> MATLAB Function3/1(seed)
  Gain1/1 -> wind y/1, Mux2/2
  Gain2/1 -> wind z/1, Mux2/3
  Demux/1 -> Gain/1
  Demux/3 -> Gain2/1
  MATLAB Function3/1(wind) -> Demux/1
  Gain/1 -> wind x/1, Mux2/1
  Mux2/1 -> wind vec/1

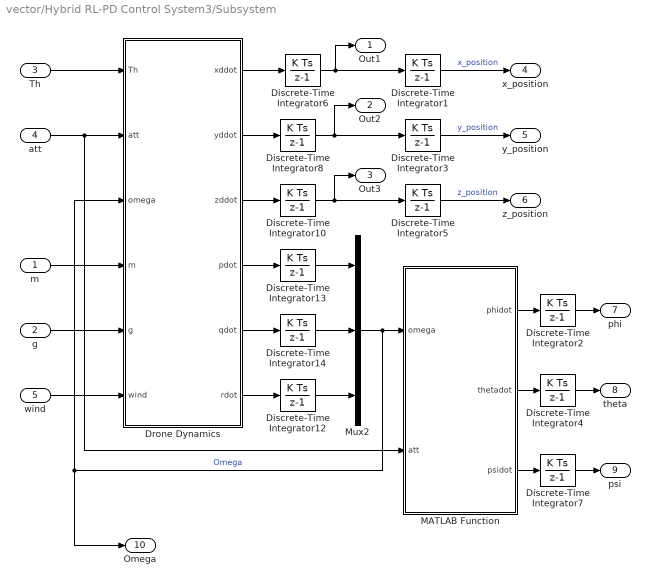
== system vector/Hybrid RL-PD Control System3/Subsystem ==
  m : Inport
  g : Inport  Port=2
  Th : Inport  Port=3
  att : Inport  Port=4
  wind : Inport  Port=5
  Discrete-Time Integrator{1..4,6..8,10,12..14} (11 alike) : DiscreteIntegrator  SampleTime=-1  ICPrevOutput=DiscIntNeverNeededParam  ICPrevScaledInput=DiscIntNeverNeededParam
  Discrete-Time Integrator5 : DiscreteIntegrator  InitialCondition=25  SampleTime=-1  ICPrevOutput=DiscIntNeverNeededParam  ICPrevScaledInput=DiscIntNeverNeededParam
  Drone Dynamics : MATLAB Function  TreatAsAtomicUnit=on
  MATLAB Function : MATLAB Function  TreatAsAtomicUnit=on
  Mux2 : Mux  Inputs=3
  Out1 : Outport
  Out2 : Outport  Port=2
  Out3 : Outport  Port=3
  x_position : Outport  Port=4
  y_position : Outport  Port=5
  z_position : Outport  Port=6
  phi : Outport  Port=7
  theta : Outport  Port=8
  psi : Outport  Port=9
  Omega : Outport  Port=10
  wires:
  Discrete-Time Integrator13/1 -> Mux2/1
  Drone Dynamics/2(yddot) -> Discrete-Time Integrator8/1
  Discrete-Time Integrator6/1 -> Out1/1, Discrete-Time Integrator1/1
  Discrete-Time Integrator10/1 -> Discrete-Time Integrator5/1, Out3/1
  Discrete-Time Integrator8/1 -> Discrete-Time Integrator3/1, Out2/1
  Th/1 -> Drone Dynamics/1(Th)
  Mux2/1 -> MATLAB Function/1(omega), Omega/1, Drone Dynamics/3(omega)  "Omega"
  Drone Dynamics/5(qdot) -> Discrete-Time Integrator14/1
  Discrete-Time Integrator14/1 -> Mux2/2
  Discrete-Time Integrator3/1 -> y_position/1  "y_position"
  MATLAB Function/2(thetadot) -> Discrete-Time Integrator4/1
  wind/1 -> Drone Dynamics/6(wind)
  MATLAB Function/3(psidot) -> Discrete-Time Integrator7/1
  m/1 -> Drone Dynamics/4(m)
  Drone Dynamics/3(zddot) -> Discrete-Time Integrator10/1
  Drone Dynamics/1(xddot) -> Discrete-Time Integrator6/1
  Drone Dynamics/4(pdot) -> Discrete-Time Integrator13/1
  Discrete-Time Integrator12/1 -> Mux2/3
  Drone Dynamics/6(rdot) -> Discrete-Time Integrator12/1
  MATLAB Function/1(phidot) -> Discrete-Time Integrator2/1
  att/1 -> MATLAB Function/2(att), Drone Dynamics/2(att)
  g/1 -> Drone Dynamics/5(g)
  Discrete-Time Integrator2/1 -> phi/1
  Discrete-Time Integrator1/1 -> x_position/1  "x_position"
  Discrete-Time Integrator7/1 -> psi/1
  Discrete-Time Integrator5/1 -> z_position/1  "z_position"
  Discrete-Time Integrator4/1 -> theta/1

== system vector/Hybrid RL-PD Control System3/Wind Subsystem ==
  Constant2 : Constant
  Product : Product
  Wind : Subsystem
  Out1 : Outport
  wires:
  Constant2/1 -> Product/1
  Wind/1(wind vec) -> Product/2  "wind vec"
  Product/1 -> Out1/1

== system vector/Reward/weight block ==
  velo : Inport
  Constant : Constant
  Dot Product : DotProduct  OutDataTypeStr=Inherit: Inherit via internal rule
  Sqrt : Sqrt
  Sum : Sum  Inputs=|++
  Tanh : Trigonometry  Operator=tanh
  k_gain : Gain  Gain=0.3
  k_gain1 : Gain  Gain=2
  weight : Outport
  wires:
  Sum/1 -> weight/1  "w_vec"
  Constant/1 -> Sum/2
  Dot Product/1 -> Sqrt/1
  Sqrt/1 -> k_gain/1
  Tanh/1 -> k_gain1/1
  k_gain/1 -> Tanh/1
  k_gain1/1 -> Sum/1
  velo/1 -> Dot Product/2, Dot Product/1

== system vector/Reward1/weight block ==
  velo : Inport
  Constant : Constant
  Dot Product : DotProduct  OutDataTypeStr=Inherit: Inherit via internal rule
  Sqrt : Sqrt
  Sum : Sum  Inputs=|++
  Tanh : Trigonometry  Operator=tanh
  k_gain : Gain  Gain=0.3
  k_gain1 : Gain  Gain=2
  weight : Outport
  wires:
  Sum/1 -> weight/1  "w_vec"
  Constant/1 -> Sum/2
  Dot Product/1 -> Sqrt/1
  Sqrt/1 -> k_gain/1
  Tanh/1 -> k_gain1/1
  k_gain/1 -> Tanh/1
  k_gain1/1 -> Sum/1
  velo/1 -> Dot Product/2, Dot Product/1

== system vector/Reward2/weight block ==
  velo : Inport
  Constant : Constant
  Dot Product : DotProduct  OutDataTypeStr=Inherit: Inherit via internal rule
  Sqrt : Sqrt
  Sum : Sum  Inputs=|++
  Tanh : Trigonometry  Operator=tanh
  k_gain : Gain  Gain=0.3
  k_gain1 : Gain  Gain=2
  weight : Outport
  wires:
  Sum/1 -> weight/1  "w_vec"
  Constant/1 -> Sum/2
  Dot Product/1 -> Sqrt/1
  Sqrt/1 -> k_gain/1
  Tanh/1 -> k_gain1/1
  k_gain/1 -> Tanh/1
  k_gain1/1 -> Sum/1
  velo/1 -> Dot Product/2, Dot Product/1

== system vector/Hybrid RL-PD Control System3/Wind Subsystem/Wind ==
  Demux : Demux  Outputs=3
  Gain : Gain  Gain=2
  Gain1 : Gain  Gain=2
  Gain2 : Gain  Gain=1.2
  MATLAB Function3 : MATLAB Function  TreatAsAtomicUnit=on
  Mux2 : Mux  Inputs=3
  Seed : Constant  Value=17119
  wind vec : Outport
  wind x : Outport  Port=2
  wind y : Outport  Port=3
  wind z : Outport  Port=4
  wires:
  Demux/2 -> Gain1/1
  Seed/1 -> MATLAB Function3/1(seed)
  Gain1/1 -> wind y/1, Mux2/2
  Gain2/1 -> wind z/1, Mux2/3
  Demux/1 -> Gain/1
  Demux/3 -> Gain2/1
  MATLAB Function3/1(wind) -> Demux/1
  Gain/1 -> wind x/1, Mux2/1
  Mux2/1 -> wind vec/1

== matlab function vector/Hybrid RL-PD Control System/Wind/MATLAB Function3 ==
  data: seed input size=[1 1]; wind output
function wind = fcn(seed)
%#codegen
% seed : scalar double
% wind : [3x1] double

    % ===== 사용자 설정 =====
    Ts    = 0.05;
    tau   = [0.8; 0.8; 1.0];
    sigma = [1.0; 1.0; 0.5];
    clip  = 6.0;

    % ===== persistent states =====
    persistent w lastSeed n
    if isempty(w)
        w = zeros(3,1);
        lastSeed = -1;
        n = 0;
    end

    % ===== seed가 바뀌면 상태 리셋 =====
    if seed ~= lastSeed
        w = zeros(3,1);
        lastSeed = seed;
        n = 0;
    end

    % ===== OU update 계수 =====
    a = exp(-Ts ./ tau);
    b = sigma .* sqrt(max(0, 1 - a.^2));

    % ===== seed 기반 의사난수 생성 =====
    % 같은 seed면 같은 순서의 z가 나옴
    z = zeros(3,1);

    for k = 1:3
        t1 = seed*12.9898 + (n+1)*78.233 + k*37.719;
        t2 = seed*39.3467 + (n+1)*11.135 + k*83.155;

        u1 = sin(t1) * 43758.5453;
        u2 = sin(t2) * 24634.6345;

        u1 = u1 - floor(u1);   % frac(u1)
        u2 = u2 - floor(u2);   % frac(u2)

        % log(0) 방지
        if u1 < 1e-12
            u1 = 1e-12;
        end

        % Box-Muller
        z(k) = sqrt(-2.0*log(u1)) * cos(2.0*pi*u2);
    end

    % ===== 상태 업데이트 =====
    w = a .* w + b .* z;
    n = n + 1;

    % ===== saturation =====
    if isfinite(clip)
        w = min(max(w, -clip), clip);
    end

    wind = w;
end

== matlab function vector/Hybrid RL-PD Control System/Commander ==
  data: select input; cmd_vec output; pos input; p_star output; B_pos input; R input
function [cmd_vec, p_star] = fcn(select, pos, B_pos, R)
    % 입력:
    %   select : 모드 선택
    %   pos    : 현재 위치 [x;y;z]
    %   B_pos  : 직선 비행 목표점
    %   R      : 원 반지름 / 8자 크기
    %
    % 출력:
    %   cmd_vec : 목표 속도 벡터 [vx; vy; vz]
    %   p_star  : 기준점(또는 목표점)

    pos = pos(:);
    B_pos = B_pos(:);

    cmd_vec = [0; 0; 0];
    p_star  = pos;

    v_max = 5;
    A_pos = [0; 0; 25];   % 기본 기준점

    % 8자 경로용 내부 파라미터
    persistent s_8;
    if isempty(s_8)
        s_8 = 0;
    end

    if select == 1 % 1) 제자리 호버링 
        target_pos = A_pos; 
        p_star = target_pos; 
        e = target_pos - pos; d = norm(e); 
        dir = e / (d + 1e-6); 
        speed_cmd = v_max * tanh(0.6 * d); 
        cmd_vec = speed_cmd * dir;
        
    elseif select == 2   % 2) A에서 B까지 이동 (직선)
        p_star = p_star_finder(A_pos, B_pos, pos);
        cmd_vec = line_vec_raw(A_pos, B_pos, pos);

    elseif select == 3   % 3) 원 비행
        z_ref = A_pos(3);
        C_pos = [A_pos(1) + R; A_pos(2); z_ref];
        [p_star, circle_dir] = circle_vec(C_pos, R, z_ref, pos);
        cmd_vec = v_max * circle_dir;

    elseif select == 4   % 4) 8자 비행 (carrot-chasing)

        % =========================================================
        % 설정
        % =========================================================
        A_8 = R;        % x 방향 크기
        B_8 = R / 2;    % y 방향 크기
        z_ref = A_pos(3);

        % 현재 가지(branch) 유지용 국소 탐색 창
        s_window = 0.08;    % 이전 s 주변 탐색 범위
        n_search = 60;      % 탐색 점 개수

        % 전방 목표점 look-ahead
        s_look = 0.04;      % 너무 작으면 흔들리고, 너무 크면 코너를 깎음

        % z 제어
        kz = 1.0;
        vz_max = 2.0;

        % =========================================================
        % 1) 이전 s_8 주변에서 국소 최근접점 탐색
        %    (전체 경로 탐색 X, 현재 가지 유지 목적)
        % =========================================================
        s_candidates = linspace(s_8 - s_window, s_8 + s_window, n_search);
        s_candidates = mod(s_candidates, 1.0);

        path_candidates = [A_pos(1) + A_8*sin(2*pi*s_candidates); ...
                           A_pos(2) + B_8*sin(4*pi*s_candidates); ...
                           z_ref * ones(1, n_search)];

        dists = sqrt(sum((path_candidates - pos).^2, 1));
        [~, idx_min] = min(dists);

        s_near = s_candidates(idx_min);

        % =========================================================
        % 2) 최근접점 p_star 계산
        % =========================================================
        p_star = [A_pos(1) + A_8*sin(2*pi*s_near); ...
                  A_pos(2) + B_8*sin(4*pi*s_near); ...
                  z_ref];

        % =========================================================
        % 3) look-ahead 목표점 p_target 계산
        % =========================================================
        s_target = mod(s_near + s_look, 1.0);

        p_target = [A_pos(1) + A_8*sin(2*pi*s_target); ...
                    A_pos(2) + B_8*sin(4*pi*s_target); ...
                    z_ref];

        % 다음 step을 위해 현재 진행률 저장
        s_8 = s_near;
        eps_val = 1e-6;
        e_xy = p_target(1:2) - pos(1:2);
        d_xy = norm(e_xy);

        v_xy = e_xy/(d_xy + eps_val);

        vz = kz * (z_ref - pos(3));
        v8 = [v_xy(1); v_xy(2); vz];
        v8_hat = v8/(norm(v8) + eps_val);
        

        cmd_vec = v_max*v8_hat; 

    else
        cmd_vec = [0; 0; 0];
        p_star  = pos;
        p_target = pos;
    end
end

== matlab function vector/Reward/e_v_dir huber ==
  data: e_v_dir input; Loss_evdir output; num input
function Loss_evdir = fcn(e_v_dir, num)

    delta = 1.2; % mode 1 기준
    % delta = 0.53; % mode 2 기준
    e_v_dir = double(e_v_dir);
    e_v_dir = e_v_dir(1);   % scalar 보장

    Loss_evdir = loss(delta, e_v_dir, num);

end

function L = loss(delta, error, num)

    if num == 1
        L = delta * abs(error);
    elseif num == 2
        L = 0.5 * error^2;
    else
        if abs(error) <= delta
            L = 0.5 * error^2;
        else
            L = delta * (abs(error) - 0.5 * delta);
        end
    end
end

== matlab function vector/Reward/MATLAB Function ==
  data: cmd_vec input; e_v_dir output; velo input; e_v_mag output
function [e_v_dir, e_v_mag] = fcn(cmd_vec, velo)

    eps_val = 1e-6;

    cmd_vec = cmd_vec(:);
    velo    = velo(:);

    cmd_mag = norm(cmd_vec);
    vel_mag = norm(velo);

    % 1) 속도 크기 오차
    e_v_mag = abs(cmd_mag - vel_mag);

    % 2) smooth normalized vectors
    cmd_hat = cmd_vec / sqrt(cmd_mag^2 + eps_val^2);
    vel_hat = velo    / sqrt(vel_mag^2 + eps_val^2);

    c = dot(cmd_hat, vel_hat);
    c = max(-1, min(1, c));

    % 기본 방향 오차
    dir_raw = 1 - c;

    % 작은 속도에서는 방향 의미를 줄이는 smooth weight
    w = (cmd_mag * vel_mag) / ((cmd_mag * vel_mag) + eps_val^2);

    e_v_dir = w * dir_raw;

end

== matlab function vector/Hybrid RL-PD Control System1/Command Conversion & Attitude PD Controller ==
  data: m input; g input; acc_cmd input; U output; att input; omega input; max_thrust output
function [U, max_thrust] = fcn(m, g, acc_cmd, att, omega)

    ax_des = acc_cmd(1);
    ay_des = acc_cmd(2);
    az_des = acc_cmd(3);

    phi   = att(1);
    theta = att(2);
    psi   = att(3);

    p = omega(1);
    q = omega(2);
    r = omega(3);

    psi_des = 0;

    max_tilt = deg2rad(30);
    max_thrust = 1.5 * m * g;
    min_thrust = 0;

    Kp_phi   = 7.0;   Kd_phi   = 0.9;
    Kp_theta = 7.0;   Kd_theta = 0.9;
    Kp_psi   = 0.5;   Kd_psi   = 0.2;

    phi_des   = ( ax_des*sin(psi) - ay_des*cos(psi) ) / g;
    theta_des = ( ax_des*cos(psi) + ay_des*sin(psi) ) / g;

    phi_des   = min(max(phi_des,   -max_tilt), max_tilt);
    theta_des = min(max(theta_des, -max_tilt), max_tilt);

    cphi = cos(phi);
    cth  = cos(theta);

    den = cphi * cth;
    den = max(den, 0.2);

    U1 = m * (g + az_des) / den;
    U1 = min(max(U1, min_thrust), max_thrust);

    e_phi   = phi_des - phi;
    e_theta = theta_des - theta;
    e_psi   = mod(psi_des - psi + pi, 2*pi) - pi;

    U2 = Kp_phi   * e_phi   - Kd_phi   * p;
    U3 = Kp_theta * e_theta - Kd_theta * q;
    U4 = Kp_psi   * e_psi   - Kd_psi   * r;

    U = [U1; U2; U3; U4];
end

== matlab function vector/Hybrid RL-PD Control System1/Reference Vector Generator ==
  data: select input; cmd_vec output; pos input; p_star output; B_pos input; R input
% Commander
% select의 명령에 따라 저장된 벡터 필드를 출력
% 1) 제자리 호버링 2) A에서 B까지 이동 3) 원 벡터
% 입력 -> 현재 위치
% 출력 -> 그 위치에서의 벡터, 항로와의 최근접점

function [cmd_vec, p_star] = fcn(select, pos, B_pos, R)

    pos = pos(:);
    B_pos = B_pos(:);

    cmd_vec = [0; 0; 0];
    p_star  = pos;

    v_max = 5;
    A_pos = [0; 0; 25];

    if select == 1   % 호버링 경우

        target_pos = A_pos;
        p_star = target_pos;

        dir = dot_vec(target_pos, pos);

        d = norm(target_pos - pos);

        k_speed = 0.6;
        speed_cmd = v_max * tanh(k_speed * d);

        cmd_vec = speed_cmd * dir;

    elseif select == 2

        p_star = p_star_finder(A_pos, B_pos, pos); 
        cmd_vec = line_vec_raw(A_pos, B_pos, pos);

    else

        C_pos = [A_pos(1) + R; A_pos(2); A_pos(3)];
        z_ref = A_pos(3);
        [p_star, circle_dir] = circle_vec(C_pos, R, z_ref, pos);

        cmd_vec = v_max * circle_dir;
    end

end

== matlab function vector/Hybrid RL-PD Control System1/Quadrotor Dynamics/Drone Dynamics ==
  data: Th input; xddot output; att input; m input; g input; wind input; yddot output; zddot output; phiddot output; thetaddot output; psiddot output
function [xddot, yddot, zddot, phiddot, thetaddot, psiddot] = fcn(Th, att, m, g, wind)

    Th1 = Th(1);
    Th2 = Th(2);
    Th3 = Th(3);
    Th4 = Th(4);

    phi   = att(1);
    theta = att(2);
    psi   = att(3);

    Fx = wind(1);
    Fy = wind(2);
    Fz = wind(3);

    % parameters
    l = 0.32;
    Ix = 0.07;
    Iy = 0.07;
    Iz = 0.12;
    kpsi = 0.05;

    % total thrust
    U1 = Th1 + Th2 + Th3 + Th4;

    % translational acceleration
    xddot = ( U1*(cos(psi)*sin(theta)*cos(phi) + sin(psi)*sin(phi)) + Fx ) / m;
    yddot = ( U1*(sin(psi)*sin(theta)*cos(phi) - cos(psi)*sin(phi)) + Fy ) / m;
    zddot = ( U1*(cos(theta)*cos(phi)) - m*g + Fz ) / m;

    % torques
    tau_phi   = (l/sqrt(2)) * (Th1 - Th2 - Th3 + Th4);
    tau_theta = (l/sqrt(2)) * (Th1 + Th2 - Th3 - Th4);
    tau_psi   = kpsi * (-Th1 + Th2 - Th3 + Th4);

    % angular acceleration (simplified)
    phiddot   = tau_phi   / Ix;
    thetaddot = tau_theta / Iy;
    psiddot   = tau_psi   / Iz;

end

== matlab function vector/Hybrid RL-PD Control System1/Thrust Mixer ==
  data: U input; Th output; max_thrust input
function Th = fcn(U, max_thrust)

    U1 = U(1);
    U2 = U(2);
    U3 = U(3);
    U4 = U(4);

    l = 0.32;          % arm length [m]
    kpsi = 0.05;      % yaw mixing gain
    Th_max = max_thrust;

    a = sqrt(2)/(4*l);

    Th1 = 0.25*U1 + a*U2 + a*U3 - kpsi*U4;
    Th2 = 0.25*U1 - a*U2 + a*U3 + kpsi*U4;
    Th3 = 0.25*U1 - a*U2 - a*U3 - kpsi*U4;
    Th4 = 0.25*U1 + a*U2 - a*U3 + kpsi*U4;

    Th1 = min(max(Th1, 0), Th_max);
    Th2 = min(max(Th2, 0), Th_max);
    Th3 = min(max(Th3, 0), Th_max);
    Th4 = min(max(Th4, 0), Th_max);

    Th = [Th1; Th2; Th3; Th4];

end

== matlab function vector/Hybrid RL-PD Control System1/Translational Controller ==
  data: acc_cmd output; cmd_vec input; vel input
% Velocity-to-Acceleration Controller
% 입력 -> 속도, 명령 벡터
% 출력 -> 가속도 벡터

function acc_cmd = fcn(cmd_vec, vel)

    x_vel = vel(1);
    y_vel = vel(2);
    z_vel = vel(3);

    % x_error = pos_error(1);
    % y_error = pos_error(2);
    % z_error = pos_error(3);
    
    xv_error = cmd_vec(1) - x_vel;
    yv_error = cmd_vec(2) - y_vel;
    zv_error = cmd_vec(3) - z_vel;

    Kp_hoz = 4.4; 
    Kp_alt = 3; 

    desired_acc_x = Kp_hoz * xv_error;
    desired_acc_y = Kp_hoz * yv_error;
    desired_acc_z = Kp_alt * zv_error;

    acc_cmd = [desired_acc_x; desired_acc_y; desired_acc_z];
    
end

== matlab function vector/Hybrid RL-PD Control System1/Wind/MATLAB Function3 ==
  data: seed input size=[1 1]; wind output
function wind = fcn(seed)
%#codegen
% seed : scalar double
% wind : [3x1] double

    % ===== 사용자 설정 =====
    Ts    = 0.01;
    tau   = [0.8; 0.8; 1.0];
    sigma = [1.0; 1.0; 0.5];
    clip  = 6.0;

    % ===== persistent states =====
    persistent w lastSeed n
    if isempty(w)
        w = zeros(3,1);
        lastSeed = -1;
        n = 0;
    end

    % ===== seed가 바뀌면 상태 리셋 =====
    if seed ~= lastSeed
        w = zeros(3,1);
        lastSeed = seed;
        n = 0;
    end

    % ===== OU update 계수 =====
    a = exp(-Ts ./ tau);
    b = sigma .* sqrt(max(0, 1 - a.^2));

    % ===== seed 기반 의사난수 생성 =====
    % 같은 seed면 같은 순서의 z가 나옴
    z = zeros(3,1);

    for k = 1:3
        t1 = seed*12.9898 + (n+1)*78.233 + k*37.719;
        t2 = seed*39.3467 + (n+1)*11.135 + k*83.155;

        u1 = sin(t1) * 43758.5453;
        u2 = sin(t2) * 24634.6345;

        u1 = u1 - floor(u1);   % frac(u1)
        u2 = u2 - floor(u2);   % frac(u2)

        % log(0) 방지
        if u1 < 1e-12
            u1 = 1e-12;
        end

        % Box-Muller
        z(k) = sqrt(-2.0*log(u1)) * cos(2.0*pi*u2);
    end

    % ===== 상태 업데이트 =====
    w = a .* w + b .* z;
    n = n + 1;

    % ===== saturation =====
    if isfinite(clip)
        w = min(max(w, -clip), clip);
    end

    wind = w;
end

== matlab function vector/Reward1/ e_angle huber ==
  data: angle_error input; Loss_phi output; Loss_theta output; Loss_psi output
function [Loss_phi, Loss_theta, Loss_psi] = fcn(angle_error)

    phi_error = angle_error(1);
    theta_error = angle_error(2);
    psi_error = mod(angle_error(3) + pi, 2*pi) - pi;

    delta = 0.21;

    if abs(phi_error) <= delta
        Loss_phi = 0.5 * phi_error^2;
    else
        Loss_phi = delta * (abs(phi_error) - 0.5 * delta);
    end

    if abs(theta_error) <= delta
        Loss_theta = 0.5 * theta_error^2;
    else
        Loss_theta = delta * (abs(theta_error) - 0.5 * delta);
    end

    if abs(psi_error) <= delta
        Loss_psi = 0.5 * psi_error^2;
    else
        Loss_psi = delta * (abs(psi_error) - 0.5 * delta);
    end

end
